simulink model "OnlyTire"  (R2021b)
settings: Solver=FixedStepAuto  StartTime=0.0  StopTime=1000  FixedStep=0.1  RelTol=1e-3
values from neighbouring files (symbols this model uses):
  g = 9.80665    [VehicleParams20_ver230707.m]
libraries: simulink x1
settings Model: Creator=tsuyoshi  LastModifiedBy=tsuyoshi

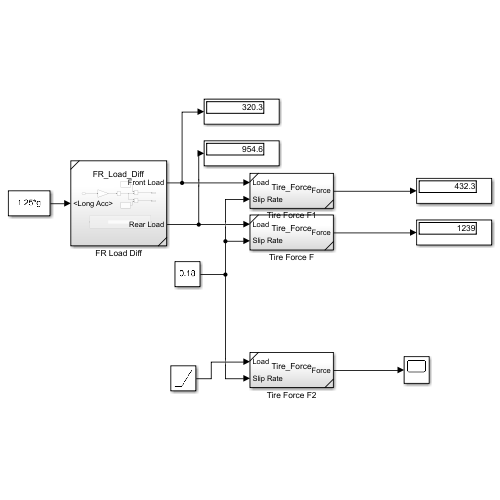
[thumbnail: Simulink's stored preview of the top-level diagram]
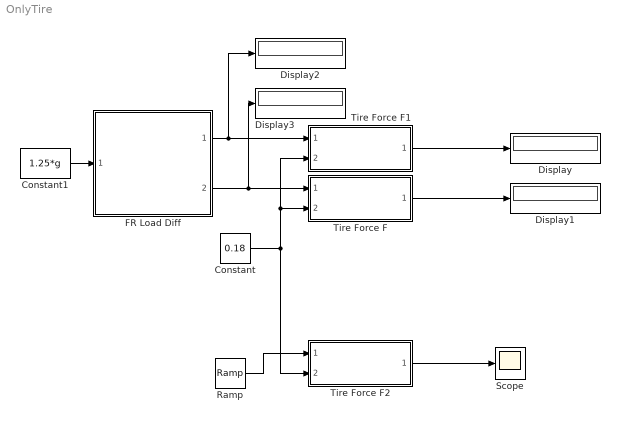
== system OnlyTire ==
  Constant : Constant  Value=0.18
  Constant1 : Constant  Value=1.25*g
  Display{,1..3} (4 alike) : Display
  FR Load Diff : Subsystem  ReferencedSubsystem=FR_Load_Diff
  Ramp : simulink/Sources/Ramp  slope=1  start=0  InitialOutput=0
  Scope : Scope
  Tire Force F : Subsystem  ReferencedSubsystem=Tire_Force
  Tire Force F1 : Subsystem  ReferencedSubsystem=Tire_Force
  Tire Force F2 : Subsystem  ReferencedSubsystem=Tire_Force
  wires:
  FR Load Diff/2 -> Display3/1, Tire Force F/1
  FR Load Diff/1 -> Display2/1, Tire Force F1/1
  Constant/1 -> Tire Force F/2, Tire Force F1/2, Tire Force F2/2
  Tire Force F1/1 -> Display/1
  Tire Force F/1 -> Display1/1
  Constant1/1 -> FR Load Diff/1
  Tire Force F2/1 -> Scope/1
  Ramp/1 -> Tire Force F2/1
